simulink model "schema_sistema_regolato"  (Simulink 7.5)
settings: Solver=ode45  StartTime=0.0  StopTime=10.0  MaxStep=0.01  RelTol=1e-3
values from neighbouring files (symbols this model uses):
  A = [0 1;-k/M -h/M]    [controllo_massa.m]
  B = [0;1/M]    [controllo_massa.m]
  C = [1 0]    [controllo_massa.m]
  D = 0    [controllo_massa.m]
  K = -place(A,B,aval_desiderati)    [controllo_massa.m]
  ueq = 3    [controllo_massa.m]
  x0 = [1;0]    [controllo_massa.m]
  xeq = [0;0]    [controllo_massa.m]
libraries: simulink x1
settings Model: Creator=professore  LastModifiedBy=professore

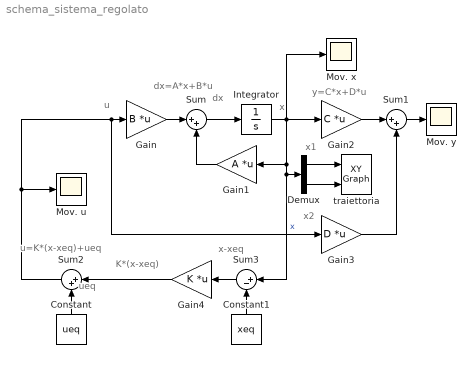
== system schema_sistema_regolato ==
  note: dx=A*x+B*u
  note: y=C*x+D*u
  note: u=K*(x-xeq)+ueq
  note: dx
  note: x
  note: u
  note: K*(x-xeq)
  note: ueq
  note: x-xeq
  note: x1
  note: x2
  Constant : Constant  Value=ueq  OutDataType=fixdt(1, 16)  OutScaling=2^0
  Constant1 : Constant  Value=xeq  OutDataType=fixdt(1, 16)  OutScaling=2^0
  Demux : Demux  Outputs=2
  Gain : Gain  Gain=B  Multiplication=Matrix(K*u)  ParameterDataType=fixdt(1, 16)  ParameterScaling=2^0  OutDataType=fixdt(1, 16)  OutScaling=2^0
  Gain1 : Gain  Gain=A  Multiplication=Matrix(K*u)  ParameterDataType=fixdt(1, 16)  ParameterScaling=2^0  OutDataType=fixdt(1, 16)  OutScaling=2^0
  Gain2 : Gain  Gain=C  Multiplication=Matrix(K*u)  ParameterDataType=fixdt(1, 16)  ParameterScaling=2^0  OutDataType=fixdt(1, 16)  OutScaling=2^0
  Gain3 : Gain  Gain=D  Multiplication=Matrix(K*u)  ParameterDataType=fixdt(1, 16)  ParameterScaling=2^0  OutDataType=fixdt(1, 16)  OutScaling=2^0
  Gain4 : Gain  Gain=K  Multiplication=Matrix(K*u)  ParameterDataType=fixdt(1, 16)  ParameterScaling=2^0  OutDataType=fixdt(1, 16)  OutScaling=2^0
  Integrator : Integrator  InitialCondition=x0
  Mov. u : Scope
      settings: SaveName=ScopeData2
  Mov. x : Scope
  Mov. y : Scope
  Sum : Sum  Inputs=|++  OutDataType=fixdt(1, 16)  OutScaling=2^0
  Sum1 : Sum  Inputs=|++  OutDataType=fixdt(1, 16)  OutScaling=2^0
  Sum2 : Sum  Inputs=|++  OutDataType=fixdt(1, 16)  OutScaling=2^0
  Sum3 : Sum  Inputs=|+-  OutDataType=fixdt(1, 16)  OutScaling=2^0
  traiettoria : simulink/Sinks/XY Graph  SystemSampleTime=-1  xmin=1  xmax=1.5  ymin=0  ymax=2  st=-1
  wires:
  Gain/1 -> Sum/1
  Gain1/1 -> Sum/2
  Sum/1 -> Integrator/1
  Integrator/1 -> Gain2/1, Gain1/1, Sum3/1, Demux/1, Mov. x/1  "x"
  Gain2/1 -> Sum1/1
  Gain3/1 -> Sum1/2
  Gain4/1 -> Sum2/1
  Constant/1 -> Sum2/2
  Sum3/1 -> Gain4/1
  Constant1/1 -> Sum3/2
  Sum2/1 -> Gain/1, Gain3/1, Mov. u/1
  Sum1/1 -> Mov. y/1
  Demux/1 -> traiettoria/1
  Demux/2 -> traiettoria/2
